simulink model "lat_accn"  (R2015a)
settings: Solver=ode3  StartTime=0.0  StopTime=12  RelTol=1e-3
settings Model: Creator=BML  LastModifiedBy=BML

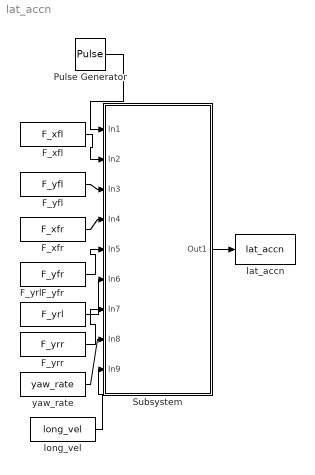
== system lat_accn ==
  F_xfl : FromWorkspace  VariableName=F_xfl  SampleTime=0
  F_xfr : FromWorkspace  VariableName=F_xfr  SampleTime=0
  F_yfl : FromWorkspace  VariableName=F_yfl  SampleTime=0
  F_yfr : FromWorkspace  VariableName=F_yfr  SampleTime=0
  F_yrl : FromWorkspace  VariableName=F_yrl  SampleTime=0
  F_yrr : FromWorkspace  VariableName=F_yrr  SampleTime=0
  Pulse Generator : DiscretePulseGenerator  PulseType=Time based  Amplitude=0  Period=8  PulseWidth=5  PhaseDelay=3
  Subsystem : Subsystem
  lat_accn : ToWorkspace  VariableName=lat_accn  SaveFormat=Timeseries  SampleTime=-1
  long_vel : FromWorkspace  VariableName=long_vel  SampleTime=0
  yaw_rate : FromWorkspace  VariableName=yaw_rate  SampleTime=0
  wires:
  Pulse Generator/1 -> Subsystem/1(In1)
  F_xfl/1 -> Subsystem/2(In2)
  F_yfl/1 -> Subsystem/3(In3)
  F_xfr/1 -> Subsystem/4(In4)
  F_yfr/1 -> Subsystem/5(In5)
  F_yrl/1 -> Subsystem/6(In6)
  F_yrr/1 -> Subsystem/7(In7)
  yaw_rate/1 -> Subsystem/8(In8)
  long_vel/1 -> Subsystem/9(In9)
  Subsystem/1(Out1) -> lat_accn/1

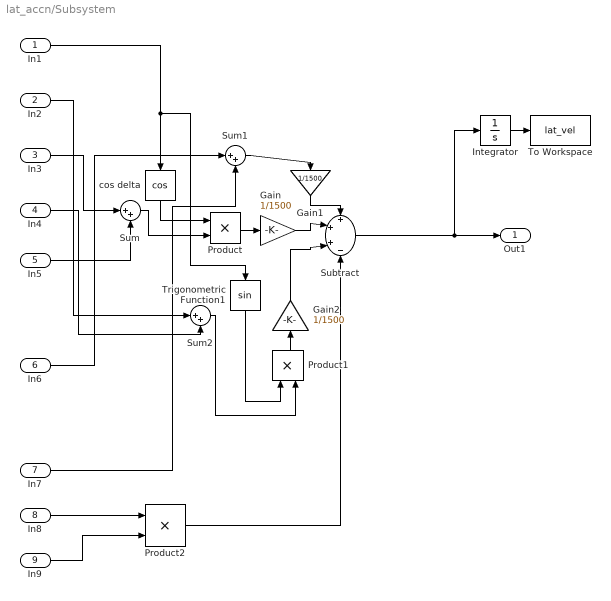
== system lat_accn/Subsystem ==
  In1 : Inport
  In2 : Inport  Port=2
  In3 : Inport  Port=3
  In4 : Inport  Port=4
  In5 : Inport  Port=5
  In6 : Inport  Port=6
  In7 : Inport  Port=7
  In8 : Inport  Port=8
  In9 : Inport  Port=9
  Gain : Gain  Gain=1/1500
  Gain1 : Gain  Gain=1/1500
  Gain2 : Gain  Gain=1/1500
  Integrator : Integrator
  Product : Product
  Product1 : Product
  Product2 : Product
  Subtract : Sum  Inputs=+++-
  Sum : Sum  Inputs=|++
  Sum1 : Sum  Inputs=|++
  Sum2 : Sum  Inputs=|++
  To Workspace : ToWorkspace  VariableName=lat_vel  SaveFormat=Timeseries  SampleTime=-1
  Trigonometric Function1 : Trigonometry
  cos delta : Trigonometry  Operator=cos
  Out1 : Outport
  wires:
  Gain/1 -> Subtract/2
  cos delta/1 -> Product/1
  Sum/1 -> Product/2
  Gain1/1 -> Subtract/1
  Sum1/1 -> Gain1/1
  In9/1 -> Product2/2
  Product/1 -> Gain/1
  In1/1 -> Trigonometric Function1/1, cos delta/1
  Trigonometric Function1/1 -> Product1/1
  Sum2/1 -> Product1/2
  Product2/1 -> Subtract/4
  Product1/1 -> Gain2/1
  In4/1 -> Sum2/2
  In2/1 -> Sum2/1
  Gain2/1 -> Subtract/3
  In5/1 -> Sum/2
  In6/1 -> Sum1/1
  In8/1 -> Product2/1
  In3/1 -> Sum/1
  In7/1 -> Sum1/2
  Subtract/1 -> Integrator/1, Out1/1
  Integrator/1 -> To Workspace/1
